simulink model "oloop1a"  (Simulink 10.0)
settings: Solver=ode15s  StartTime=0.0  StopTime=120  MaxStep=2  RelTol=1e-3  AbsTol=1e-3
undefined symbols (not defined in the file): uaero0, uprop0
libraries: fdclib10 x1, simulink3 x1
settings Model: Creator=bhisma  LastModifiedBy=bhisma  ExtModeTrigMode=oneshot  ExtModeArmWhenConnect=off
settings DataIOCC: SignalLoggingSaveFormat=ModelDataLogs  SaveOutput=off  SaveTime=off
settings OptimizationCC: BlockReduction=off  BooleanDataType=off  LifeSpan=auto
settings DebuggingCC: SaveWithParameterizedLinksMsg=none  SignalResolutionControl=TryResolveAllWithWarning  MultiTaskDSMMsg=warning  MultiTaskCondExecSysMsg=none  SFUnexpectedBacktrackingDiag=error  SFNoUnconditionalDefaultTransitionDiag=error  SFExecutionAtInitializationDiag=warning  ArithmeticOperatorsInVariantConditions=error
settings HardwareCC: ProdBitPerPointer=64  ProdBitPerSizeT=64  ProdBitPerPtrDiffT=64  ProdLargestAtomicFloat=Float  ProdIntDivRoundTo=Zero  ProdEndianess=LittleEndian  ProdWordSize=64  ProdHWDeviceType=Intel->x86-64 (Windows64)  TargetUnknown=on
settings SFSimCC: SimUseLocalCustomCode=on  CustomCodeUndefinedFunction=FilterOut
settings RTWCC: TemplateMakefile=grt_vc.tmf  RTWUseLocalCustomCode=on
settings CodeAppCC: StateflowObjectComments=off
settings GRTTargetCC: TargetLangStandard=C99 (ISO)
settings ConfigComp: CovMetricSettings=dwe  CovHtmlReporting=off  CovSaveCumulativeToWorkspaceVar=off  CovSaveSingleToWorkspaceVar=off

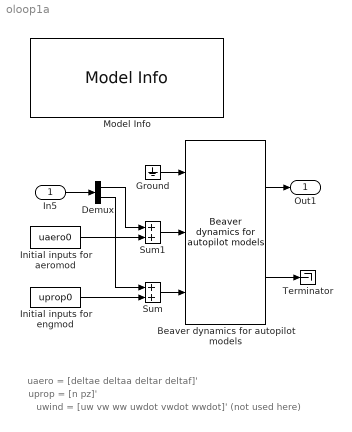
== system oloop1a ==
  note: uaero = [deltae deltaa deltar deltaf]'
  note: uprop = [n pz]'
  note: uwind = [uw vw ww uwdot vwdot wwdot]' (not used here)
  In5 : Inport
  Beaver dynamics for autopilot models : fdclib10/Beaver dynamics for autopilot models
  Demux : Demux  Outputs=[4 2]
  Ground : Ground
  Initial inputs for aeromod : Constant  Value=uaero0
  Initial inputs for engmod : Constant  Value=uprop0
  Model Info : simulink3/Signals & Systems/Model Info  InitialBlockCM=none  BlockCM=none  Frame=on  DisplayStringWithTags=|  HorizontalTextAlignment=Center  LeftAlignmentValue=0.5  SourceBlockDiagram=oloop1a  TagMaxNumber=20
      | Test system to validate nonlinear
      | open-loop simulations of the 'Beaver'.
      | Used by OPENLOOP.M.
      | 
      | M.O. Rauw, March 2004
      settings: SourceProductName=Simulink  SourceProductBaseCode=SL
  Sum : Sum  SaturateOnIntegerOverflow=on  InputSameDT=on  OutDataTypeStr=Inherit: Same as first input
  Sum1 : Sum  SaturateOnIntegerOverflow=on  InputSameDT=on  OutDataTypeStr=Inherit: Same as first input
  Terminator : Terminator
  Out1 : Outport
  wires:
  Sum1/1 -> Beaver dynamics for autopilot models/2
  Sum/1 -> Beaver dynamics for autopilot models/3
  Beaver dynamics for autopilot models/1 -> Out1/1
  Beaver dynamics for autopilot models/2 -> Terminator/1
  Ground/1 -> Beaver dynamics for autopilot models/1
  Initial inputs for aeromod/1 -> Sum1/2
  Initial inputs for engmod/1 -> Sum/2
  Demux/2 -> Sum/1
  Demux/1 -> Sum1/1
  In5/1 -> Demux/1
